simulink model "W01_Base_Map_cs"  (R2019a)
settings: Solver=FixedStepDiscrete  StartTime=0.0  StopTime=inf  FixedStep=1/20  RelTol=1e-3
PreLoadFcn:
  | mbxruntime.callbacks.PreLoadFcn(bdroot);
  | check_NUTS_defined
  | model_closed = 0;
  | assignin('base',['model_closed_' bdroot],false);
PostLoadFcn:
  | mbxruntime.callbacks.PostLoadFcn(bdroot);
InitFcn:
  | mbxruntime.callbacks.InitFcn(bdroot);
StartFcn:
  | mbxruntime.callbacks.StartFcn(bdroot);
StopFcn:
  | mbxruntime.callbacks.StopFcn(bdroot);;
  | 
model workspace: external: MAT-File .\W01_Base_Map_cs_hws.mat (data not in the file)
undefined symbols (not defined in the file or in its folder): DiscIntNeverNeededParam, Header, InitImageOutputDir, mbxruntime, Poses, Poses_SL_Info, tabledata, W01_Base_Map_cs_004987d4dd39f9b6, W01_Base_Map_cs_00cc66853e964a64, W01_Base_Map_cs_00f75b713170549a, W01_Base_Map_cs_01472650a6655f66, W01_Base_Map_cs_021eada97d6d5412, W01_Base_Map_cs_0288936122941f67, W01_Base_Map_cs_03728bc5c0f611d1, W01_Base_Map_cs_03729b7883682eca, W01_Base_Map_cs_03935175e827b825, W01_Base_Map_cs_03ecb5a7ceaf36f1, W01_Base_Map_cs_04544dd62153117c, W01_Base_Map_cs_04f0838a8dce3a91, W01_Base_Map_cs_05c6883b663017e6, W01_Base_Map_cs_074ff6b44c8e4b42, W01_Base_Map_cs_0850adb5f9b52847, W01_Base_Map_cs_09b4416d284a38c0, W01_Base_Map_cs_09f1a8cccf5dc476, W01_Base_Map_cs_0a863e6a78242047, W01_Base_Map_cs_0b51b2edfb6b21eb, W01_Base_Map_cs_0c25b2d8edd3fbea, W01_Base_Map_cs_0cec291d859792a3, W01_Base_Map_cs_0d48999ceb9def0a, W01_Base_Map_cs_1054e386bc2b89f8, W01_Base_Map_cs_129d7fd29679c9e4, W01_Base_Map_cs_1557dafebe6eb5e3, W01_Base_Map_cs_155bf6da17508b9f, W01_Base_Map_cs_1619aae3285d69a6, W01_Base_Map_cs_18faf784f59d6ded, W01_Base_Map_cs_190ae931cd3b3df1, W01_Base_Map_cs_1a47612a95ab18a1, W01_Base_Map_cs_1a96581334d27a16, W01_Base_Map_cs_1b9c28e1ad91b987, W01_Base_Map_cs_1bd80946b29cc249, W01_Base_Map_cs_1bf8c5472ecd97cc, W01_Base_Map_cs_1c047b8f6e9a46e9, W01_Base_Map_cs_1c4e91c4c8848966, W01_Base_Map_cs_1dfe629d3c3a34d6, W01_Base_Map_cs_1e00e80d4fa95f87, W01_Base_Map_cs_1e67a7d0e7e33a10, W01_Base_Map_cs_1e994bb86296e53e, W01_Base_Map_cs_1f3d28b65a209a81, W01_Base_Map_cs_1f4ddfcaed2bdfa2, W01_Base_Map_cs_20e6a062a8bf989a, W01_Base_Map_cs_210ba2feda70a68e, W01_Base_Map_cs_211f71a4af886b52, W01_Base_Map_cs_2177d1459a678375, W01_Base_Map_cs_21a90c8036f5a434, W01_Base_Map_cs_230365adf03440eb, W01_Base_Map_cs_2309b1b7588d9eb5, W01_Base_Map_cs_25766054964f8b23, W01_Base_Map_cs_25e42a2c513fe98c, W01_Base_Map_cs_25e53e1123ccd658, W01_Base_Map_cs_263f0dd851f19fdf ... (+283)
libraries: PreScanSimulinkLibrary x112, robotcorelib x55, adeye_lib x46, simulink x31, simulink_extras x24, robotlib x3, PreScanUsefulBlocks x1
(part 21 of 32)

== system W01_Base_Map_cs/Male_LargeShoulderSuitcase_1/SELF_Demux ==
  SELF : Inport  OutDataTypeStr=Bus: PRESCAN_SELFSENSORDATA
  Bus Selector : BusSelector  OutputSignals=PositionX,PositionY,PositionZ,OrientationRoll,OrientationPitch,OrientationYaw,Velocity,Yaw_rate,Lat,Long,Alt,TimeStamp
  Demux2 : Demux  Outputs=3
  Gain : Gain  Gain=180/pi
  Gain1 : Gain  Gain=180/pi
  Vector Concatenate1 : Concatenate  NumInputs=3
  compas converter : Subsystem
  x [m] : Outport
  y [m] : Outport  Port=2
  z [m] : Outport  Port=3
  rotx [deg] : Outport  Port=4
  roty [deg] : Outport  Port=5
  rotz [deg] : Outport  Port=6
  GPS lat [deg] : Outport  Port=7
  GPS long [deg] : Outport  Port=8
  GPS alt [m] : Outport  Port=9
  velocity [m/s] : Outport  Port=10
  heading [deg] : Outport  Port=11
  yaw rate [deg/s] : Outport  Port=12
  TimeStamp [s] : Outport  Port=13
  wires:
  Bus Selector/12 -> TimeStamp [s]/1  "<TimeStamp>"
  Bus Selector/11 -> GPS alt [m]/1  "<Alt>"
  Bus Selector/10 -> GPS long [deg]/1  "<Long>"
  Bus Selector/9 -> GPS lat [deg]/1  "<Lat>"
  Bus Selector/8 -> Gain1/1  "<Yaw_rate>"
  Bus Selector/7 -> velocity [m/s]/1  "<Velocity>"
  Bus Selector/6 -> compas converter/1(rotz [rad]), Vector Concatenate1/3  "<OrientationYaw>"
  Bus Selector/5 -> Vector Concatenate1/2  "<OrientationPitch>"
  Bus Selector/4 -> Vector Concatenate1/1  "<OrientationRoll>"
  Vector Concatenate1/1 -> Gain/1
  Bus Selector/3 -> z [m]/1  "<PositionZ>"
  Bus Selector/2 -> y [m]/1  "<PositionY>"
  Bus Selector/1 -> x [m]/1  "<PositionX>"
  SELF/1 -> Bus Selector/1
  Gain/1 -> Demux2/1
  Demux2/1 -> rotx [deg]/1
  Demux2/2 -> roty [deg]/1
  Demux2/3 -> rotz [deg]/1
  compas converter/1(heading [deg]) -> heading [deg]/1
  Gain1/1 -> yaw rate [deg/s]/1

== system W01_Base_Map_cs/Male_LargeShoulderSuitcase_1/VISUColorRegion_Bag_Mux ==
  RGB [-,-,-] : Inport
  Bus Creator : BusCreator  Inputs=4  OutDataTypeStr=Bus: PRESCAN_COLOR_DATA  NonVirtualBus=on
  Constant : Constant  Value=255  OutDataTypeStr=uint8
  Data Type Conversion : DataTypeConversion  OutDataTypeStr=uint8
  Data Type Conversion1 : DataTypeConversion  OutDataTypeStr=uint8
  Data Type Conversion2 : DataTypeConversion  OutDataTypeStr=uint8
  Demux : Demux  Outputs=3
  ColorRegion : Outport  OutDataTypeStr=Bus: PRESCAN_COLOR_DATA  PortDimensions=1
  wires:
  Constant/1 -> Bus Creator/4  "A"
  Data Type Conversion2/1 -> Bus Creator/3  "B"
  Data Type Conversion1/1 -> Bus Creator/2  "G"
  Data Type Conversion/1 -> Bus Creator/1  "R"
  Demux/3 -> Data Type Conversion2/1  "B"
  Demux/2 -> Data Type Conversion1/1  "G"
  Demux/1 -> Data Type Conversion/1  "R"
  RGB [-,-,-]/1 -> Demux/1
  Bus Creator/1 -> ColorRegion/1

== system W01_Base_Map_cs/Male_LargeShoulderSuitcase_1/VISUColorRegion_Lower_Body_Mux ==
  RGB [-,-,-] : Inport
  Bus Creator : BusCreator  Inputs=4  OutDataTypeStr=Bus: PRESCAN_COLOR_DATA  NonVirtualBus=on
  Constant : Constant  Value=255  OutDataTypeStr=uint8
  Data Type Conversion : DataTypeConversion  OutDataTypeStr=uint8
  Data Type Conversion1 : DataTypeConversion  OutDataTypeStr=uint8
  Data Type Conversion2 : DataTypeConversion  OutDataTypeStr=uint8
  Demux : Demux  Outputs=3
  ColorRegion : Outport  OutDataTypeStr=Bus: PRESCAN_COLOR_DATA  PortDimensions=1
  wires:
  Constant/1 -> Bus Creator/4  "A"
  Data Type Conversion2/1 -> Bus Creator/3  "B"
  Data Type Conversion1/1 -> Bus Creator/2  "G"
  Data Type Conversion/1 -> Bus Creator/1  "R"
  Demux/3 -> Data Type Conversion2/1  "B"
  Demux/2 -> Data Type Conversion1/1  "G"
  Demux/1 -> Data Type Conversion/1  "R"
  RGB [-,-,-]/1 -> Demux/1
  Bus Creator/1 -> ColorRegion/1

== system W01_Base_Map_cs/Male_LargeShoulderSuitcase_1/VISUColorRegion_Shoes_Mux ==
  RGB [-,-,-] : Inport
  Bus Creator : BusCreator  Inputs=4  OutDataTypeStr=Bus: PRESCAN_COLOR_DATA  NonVirtualBus=on
  Constant : Constant  Value=255  OutDataTypeStr=uint8
  Data Type Conversion : DataTypeConversion  OutDataTypeStr=uint8
  Data Type Conversion1 : DataTypeConversion  OutDataTypeStr=uint8
  Data Type Conversion2 : DataTypeConversion  OutDataTypeStr=uint8
  Demux : Demux  Outputs=3
  ColorRegion : Outport  OutDataTypeStr=Bus: PRESCAN_COLOR_DATA  PortDimensions=1
  wires:
  Constant/1 -> Bus Creator/4  "A"
  Data Type Conversion2/1 -> Bus Creator/3  "B"
  Data Type Conversion1/1 -> Bus Creator/2  "G"
  Data Type Conversion/1 -> Bus Creator/1  "R"
  Demux/3 -> Data Type Conversion2/1  "B"
  Demux/2 -> Data Type Conversion1/1  "G"
  Demux/1 -> Data Type Conversion/1  "R"
  RGB [-,-,-]/1 -> Demux/1
  Bus Creator/1 -> ColorRegion/1

== system W01_Base_Map_cs/Male_LargeShoulderSuitcase_1/VISUColorRegion_Upper_body_Mux ==
  RGB [-,-,-] : Inport
  Bus Creator : BusCreator  Inputs=4  OutDataTypeStr=Bus: PRESCAN_COLOR_DATA  NonVirtualBus=on
  Constant : Constant  Value=255  OutDataTypeStr=uint8
  Data Type Conversion : DataTypeConversion  OutDataTypeStr=uint8
  Data Type Conversion1 : DataTypeConversion  OutDataTypeStr=uint8
  Data Type Conversion2 : DataTypeConversion  OutDataTypeStr=uint8
  Demux : Demux  Outputs=3
  ColorRegion : Outport  OutDataTypeStr=Bus: PRESCAN_COLOR_DATA  PortDimensions=1
  wires:
  Constant/1 -> Bus Creator/4  "A"
  Data Type Conversion2/1 -> Bus Creator/3  "B"
  Data Type Conversion1/1 -> Bus Creator/2  "G"
  Data Type Conversion/1 -> Bus Creator/1  "R"
  Demux/3 -> Data Type Conversion2/1  "B"
  Demux/2 -> Data Type Conversion1/1  "G"
  Demux/1 -> Data Type Conversion/1  "R"
  RGB [-,-,-]/1 -> Demux/1
  Bus Creator/1 -> ColorRegion/1

== system W01_Base_Map_cs/Male_Old_White_WithStick_1/Dynamics_Empty ==
  note: For state mode 'Dynamic' positions
      | are not taken into account, as they
      | are computed by integrating velocity.
      | Click annotation for Help.
  In1 : Inport
  Bus Creator : BusCreator  Inputs=3
  Bus Creator1 : BusCreator  Inputs=4
  Bus Selector : BusSelector  OutputSignals=signal1,signal2,signal3
  Bus Selector1 : BusSelector  OutputSignals=Pose.Position.X,Pose.Position.Y,Pose.Position.Z,Pose.Orientation.W,Pose.Orientation.X,Pose.Orientation.Y,Pose.Orientation.Z
  Bus to Vector : BusToVector
  Coordinate Transformation Conversion : robotcorelib/Coordinate Transformation Conversion  InputRepresentation=Quaternion  InputEulerSequence=ZYX  ShowTrVecInputPort=on  OutputRepresentation=Euler Angles  OutputEulerSequence=ZYX  ShowTrVecOutputPort=on  SimulateUsing=Interpreted execution
      settings: SourceProductBaseCode=RO
  Demux : Demux  Outputs=3
  Display{,1..3} (4 alike) : Display
  Ground_2 : Ground
  Ground_3 : Ground
  Ground_4 : Ground
  MuxState : Subsystem  Tag=mux/State  mask(Empty Dynamics State Block){positioningmode=on, TimeStep=1/20}
      mask prompts: positioningmode "Positioning Mode"; TimeStep "Auto Assigned: Time Step [s]"
      mask help:
      | Build the state of an actor based on user input.
      | The user can either use positioning mode or dynamics mode.
      | - When using positioning mode the position and orientation of the actor are set directly based on the input. Expected input is relative to the initial position and orientation of the actor. It's also possible to specify the velocity of the actor, though this input isn't used, only passed on.
      | - When using dynamics mode the position input is ignored. Expected input is velocity and orientation. The velocity is relative the current orientation of the actor, while orientation is relative to its initial orientation. The position of the actor is calculated based on the velocity and orientation given.
      settings: DeleteFcn=PreScanBlockDeleteFcn;
  STATE_Male_Old_White_WithStick_1 : Subsystem  Tag=mux/StatePort  Priority=0  LoadFcn=load PrescanStateActuatorData  mask(PreScan Sink Block: State){x0=W01_Base_Map_cs_cc1dceb6bcb11776, y0=W01_Base_Map_cs_dd1c45dbea022fa7, z0=W01_Base_Map_cs_395a0412cd743ae4, Roll0=W01_Base_Map_cs_f8d27bdcf4af038a, Pitch0=W01_Base_Map_cs_2bee40668d322807, Yaw0=W01_Base_Map_cs_3225b4cbe8940148, TimeStep=1/20}
      mask prompts: x0 "Ini x-position VEHICLE wrt GLOBAL axis system [m]"; y0 "Ini y-position VEHICLE wrt GLOBAL axis system [m]"; z0 "Ini z-position VEHICLE wrt GLOBAL axis system [m]"; Roll0 "Ini roll-angle BODY wrt VEHICLE axis system [deg]"; Pitch0 "Ini pitch-angle BODY wrt VEHICLE axis system [deg]"; Yaw0 "Ini yaw-angle VEHICLE wrt GLOBAL axis system [deg]"; TimeStep "Auto-Assigned: Upload Period [s]"
      mask help:
      | The Actor State contains a vector signal of size (9x1), containing the following signals:
      |
      | -  Position                  (x,y,z)                                     [m]
      | -  Velocity                  (vx,vy,vz)                               [m/s]
      | -  Angles                    (Roll, Pitch, Yaw)                   [rad]
      |
      | The Actor state is defined in the global axis system.
      | The state is superponed on the Initial position defined in the GUI.
      |
      | For more information, please click Help.
      settings: DeleteFcn=PreScanBlockDeleteFcn;
      mask Help: eval('openHelp(222)')
      mask Display: image(imread('State.png'))
  To Virtual Bus : SignalConversion  ConversionOutput=Virtual bus  OverrideOpt=off
  State : Outport  Tag=outport/StateOutport  SampleTime=1/20
  wires:
  MuxState/1(state) -> STATE_Male_Old_White_WithStick_1/1(State)
  STATE_Male_Old_White_WithStick_1/1(StateBus) -> State/1
  Ground_2/1 -> MuxState/4(dx [m/s])
  Ground_3/1 -> MuxState/5(dy [m/s])
  Ground_4/1 -> MuxState/6(dz [m/s])
  Bus Selector/2 -> MuxState/8(P [rad]), Display/1  "<signal2>"
  Bus Selector/1 -> MuxState/7(R [rad]), Display2/1  "<signal1>"
  Bus Selector1/2 -> MuxState/2(y [m])  "<Y>"
  Bus Selector1/1 -> MuxState/1(x [m])  "<X>"
  Coordinate Transformation Conversion/1 -> Demux/1
  Demux/1 -> Bus Creator/1
  To Virtual Bus/1 -> Bus to Vector/1
  In1/1 -> Bus Selector1/1
  Bus to Vector/1 -> Display3/1, Coordinate Transformation Conversion/1
  Bus Creator1/1 -> To Virtual Bus/1
  Demux/2 -> Bus Creator/2
  Demux/3 -> Bus Creator/3
  Bus Creator/1 -> Bus Selector/1
  Bus Selector1/7 -> Bus Creator1/4  "<Z>"
  Bus Selector1/4 -> Bus Creator1/1  "<W>"
  Bus Selector/3 -> MuxState/9(Y [rad]), Display1/1  "<signal3>"
  Bus Selector1/5 -> Bus Creator1/2  "<X>"
  Bus Selector1/3 -> MuxState/3(z [m])  "<Z>"
  Bus Selector1/6 -> Bus Creator1/3  "<Y>"

== system W01_Base_Map_cs/Male_Old_White_WithStick_1/SELF_Demux ==
  SELF : Inport  OutDataTypeStr=Bus: PRESCAN_SELFSENSORDATA
  Bus Selector : BusSelector  OutputSignals=PositionX,PositionY,PositionZ,OrientationRoll,OrientationPitch,OrientationYaw,Velocity,Yaw_rate,Lat,Long,Alt,TimeStamp
  Demux2 : Demux  Outputs=3
  Gain : Gain  Gain=180/pi
  Gain1 : Gain  Gain=180/pi
  Vector Concatenate1 : Concatenate  NumInputs=3
  compas converter : Subsystem
  x [m] : Outport
  y [m] : Outport  Port=2
  z [m] : Outport  Port=3
  rotx [deg] : Outport  Port=4
  roty [deg] : Outport  Port=5
  rotz [deg] : Outport  Port=6
  GPS lat [deg] : Outport  Port=7
  GPS long [deg] : Outport  Port=8
  GPS alt [m] : Outport  Port=9
  velocity [m/s] : Outport  Port=10
  heading [deg] : Outport  Port=11
  yaw rate [deg/s] : Outport  Port=12
  TimeStamp [s] : Outport  Port=13
  wires:
  Bus Selector/12 -> TimeStamp [s]/1  "<TimeStamp>"
  Bus Selector/11 -> GPS alt [m]/1  "<Alt>"
  Bus Selector/10 -> GPS long [deg]/1  "<Long>"
  Bus Selector/9 -> GPS lat [deg]/1  "<Lat>"
  Bus Selector/8 -> Gain1/1  "<Yaw_rate>"
  Bus Selector/7 -> velocity [m/s]/1  "<Velocity>"
  Bus Selector/6 -> compas converter/1(rotz [rad]), Vector Concatenate1/3  "<OrientationYaw>"
  Bus Selector/5 -> Vector Concatenate1/2  "<OrientationPitch>"
  Bus Selector/4 -> Vector Concatenate1/1  "<OrientationRoll>"
  Vector Concatenate1/1 -> Gain/1
  Bus Selector/3 -> z [m]/1  "<PositionZ>"
  Bus Selector/2 -> y [m]/1  "<PositionY>"
  Bus Selector/1 -> x [m]/1  "<PositionX>"
  SELF/1 -> Bus Selector/1
  Gain/1 -> Demux2/1
  Demux2/1 -> rotx [deg]/1
  Demux2/2 -> roty [deg]/1
  Demux2/3 -> rotz [deg]/1
  compas converter/1(heading [deg]) -> heading [deg]/1
  Gain1/1 -> yaw rate [deg/s]/1

== system W01_Base_Map_cs/Male_Old_White_WithStick_1/VISUColorRegion_Lower_Body_Mux ==
  RGB [-,-,-] : Inport
  Bus Creator : BusCreator  Inputs=4  OutDataTypeStr=Bus: PRESCAN_COLOR_DATA  NonVirtualBus=on
  Constant : Constant  Value=255  OutDataTypeStr=uint8
  Data Type Conversion : DataTypeConversion  OutDataTypeStr=uint8
  Data Type Conversion1 : DataTypeConversion  OutDataTypeStr=uint8
  Data Type Conversion2 : DataTypeConversion  OutDataTypeStr=uint8
  Demux : Demux  Outputs=3
  ColorRegion : Outport  OutDataTypeStr=Bus: PRESCAN_COLOR_DATA  PortDimensions=1
  wires:
  Constant/1 -> Bus Creator/4  "A"
  Data Type Conversion2/1 -> Bus Creator/3  "B"
  Data Type Conversion1/1 -> Bus Creator/2  "G"
  Data Type Conversion/1 -> Bus Creator/1  "R"
  Demux/3 -> Data Type Conversion2/1  "B"
  Demux/2 -> Data Type Conversion1/1  "G"
  Demux/1 -> Data Type Conversion/1  "R"
  RGB [-,-,-]/1 -> Demux/1
  Bus Creator/1 -> ColorRegion/1

== system W01_Base_Map_cs/Male_Old_White_WithStick_1/VISUColorRegion_Shoes_Mux ==
  RGB [-,-,-] : Inport
  Bus Creator : BusCreator  Inputs=4  OutDataTypeStr=Bus: PRESCAN_COLOR_DATA  NonVirtualBus=on
  Constant : Constant  Value=255  OutDataTypeStr=uint8
  Data Type Conversion : DataTypeConversion  OutDataTypeStr=uint8
  Data Type Conversion1 : DataTypeConversion  OutDataTypeStr=uint8
  Data Type Conversion2 : DataTypeConversion  OutDataTypeStr=uint8
  Demux : Demux  Outputs=3
  ColorRegion : Outport  OutDataTypeStr=Bus: PRESCAN_COLOR_DATA  PortDimensions=1
  wires:
  Constant/1 -> Bus Creator/4  "A"
  Data Type Conversion2/1 -> Bus Creator/3  "B"
  Data Type Conversion1/1 -> Bus Creator/2  "G"
  Data Type Conversion/1 -> Bus Creator/1  "R"
  Demux/3 -> Data Type Conversion2/1  "B"
  Demux/2 -> Data Type Conversion1/1  "G"
  Demux/1 -> Data Type Conversion/1  "R"
  RGB [-,-,-]/1 -> Demux/1
  Bus Creator/1 -> ColorRegion/1

== system W01_Base_Map_cs/Male_Old_White_WithStick_1/VISUColorRegion_Upper_Body_Mux ==
  RGB [-,-,-] : Inport
  Bus Creator : BusCreator  Inputs=4  OutDataTypeStr=Bus: PRESCAN_COLOR_DATA  NonVirtualBus=on
  Constant : Constant  Value=255  OutDataTypeStr=uint8
  Data Type Conversion : DataTypeConversion  OutDataTypeStr=uint8
  Data Type Conversion1 : DataTypeConversion  OutDataTypeStr=uint8
  Data Type Conversion2 : DataTypeConversion  OutDataTypeStr=uint8
  Demux : Demux  Outputs=3
  ColorRegion : Outport  OutDataTypeStr=Bus: PRESCAN_COLOR_DATA  PortDimensions=1
  wires:
  Constant/1 -> Bus Creator/4  "A"
  Data Type Conversion2/1 -> Bus Creator/3  "B"
  Data Type Conversion1/1 -> Bus Creator/2  "G"
  Data Type Conversion/1 -> Bus Creator/1  "R"
  Demux/3 -> Data Type Conversion2/1  "B"
  Demux/2 -> Data Type Conversion1/1  "G"
  Demux/1 -> Data Type Conversion/1  "R"
  RGB [-,-,-]/1 -> Demux/1
  Bus Creator/1 -> ColorRegion/1

== system W01_Base_Map_cs/Male_Old_White_WithWalkerWithWheels_1/Dynamics_Empty ==
  note: For state mode 'Dynamic' positions
      | are not taken into account, as they
      | are computed by integrating velocity.
      | Click annotation for Help.
  In1 : Inport
  Bus Creator : BusCreator  Inputs=3
  Bus Creator1 : BusCreator  Inputs=4
  Bus Selector : BusSelector  OutputSignals=signal1,signal2,signal3
  Bus Selector1 : BusSelector  OutputSignals=Pose.Position.X,Pose.Position.Y,Pose.Position.Z,Pose.Orientation.W,Pose.Orientation.X,Pose.Orientation.Y,Pose.Orientation.Z
  Bus to Vector : BusToVector
  Coordinate Transformation Conversion : robotcorelib/Coordinate Transformation Conversion  InputRepresentation=Quaternion  InputEulerSequence=ZYX  ShowTrVecInputPort=on  OutputRepresentation=Euler Angles  OutputEulerSequence=ZYX  ShowTrVecOutputPort=on  SimulateUsing=Interpreted execution
      settings: SourceProductBaseCode=RO
  Demux : Demux  Outputs=3
  Display{,1..3} (4 alike) : Display
  Ground_2 : Ground
  Ground_3 : Ground
  Ground_4 : Ground
  MuxState : Subsystem  Tag=mux/State  mask(Empty Dynamics State Block){positioningmode=on, TimeStep=1/20}
      mask prompts: positioningmode "Positioning Mode"; TimeStep "Auto Assigned: Time Step [s]"
      mask help:
      | Build the state of an actor based on user input.
      | The user can either use positioning mode or dynamics mode.
      | - When using positioning mode the position and orientation of the actor are set directly based on the input. Expected input is relative to the initial position and orientation of the actor. It's also possible to specify the velocity of the actor, though this input isn't used, only passed on.
      | - When using dynamics mode the position input is ignored. Expected input is velocity and orientation. The velocity is relative the current orientation of the actor, while orientation is relative to its initial orientation. The position of the actor is calculated based on the velocity and orientation given.
      settings: DeleteFcn=PreScanBlockDeleteFcn;
  STATE_Male_Old_White_WithWalkerWithWheels_1 : Subsystem  Tag=mux/StatePort  Priority=0  LoadFcn=load PrescanStateActuatorData  mask(PreScan Sink Block: State){x0=W01_Base_Map_cs_55eb73129df87210, y0=W01_Base_Map_cs_bf64c7ba95b0aa28, z0=W01_Base_Map_cs_34d2d6374cf9c3dd, Roll0=W01_Base_Map_cs_01472650a6655f66, Pitch0=W01_Base_Map_cs_7cad10af2de5dd89, Yaw0=W01_Base_Map_cs_fd671e9618ff8c80, TimeStep=1/20}
      mask prompts: x0 "Ini x-position VEHICLE wrt GLOBAL axis system [m]"; y0 "Ini y-position VEHICLE wrt GLOBAL axis system [m]"; z0 "Ini z-position VEHICLE wrt GLOBAL axis system [m]"; Roll0 "Ini roll-angle BODY wrt VEHICLE axis system [deg]"; Pitch0 "Ini pitch-angle BODY wrt VEHICLE axis system [deg]"; Yaw0 "Ini yaw-angle VEHICLE wrt GLOBAL axis system [deg]"; TimeStep "Auto-Assigned: Upload Period [s]"
      mask help:
      | The Actor State contains a vector signal of size (9x1), containing the following signals:
      |
      | -  Position                  (x,y,z)                                     [m]
      | -  Velocity                  (vx,vy,vz)                               [m/s]
      | -  Angles                    (Roll, Pitch, Yaw)                   [rad]
      |
      | The Actor state is defined in the global axis system.
      | The state is superponed on the Initial position defined in the GUI.
      |
      | For more information, please click Help.
      settings: DeleteFcn=PreScanBlockDeleteFcn;
      mask Help: eval('openHelp(222)')
      mask Display: image(imread('State.png'))
  To Virtual Bus : SignalConversion  ConversionOutput=Virtual bus  OverrideOpt=off
  State : Outport  Tag=outport/StateOutport  SampleTime=1/20
  wires:
  MuxState/1(state) -> STATE_Male_Old_White_WithWalkerWithWheels_1/1(State)
  STATE_Male_Old_White_WithWalkerWithWheels_1/1(StateBus) -> State/1
  Ground_2/1 -> MuxState/4(dx [m/s])
  Ground_3/1 -> MuxState/5(dy [m/s])
  Ground_4/1 -> MuxState/6(dz [m/s])
  Bus Selector/2 -> MuxState/8(P [rad]), Display/1  "<signal2>"
  Bus Selector/1 -> MuxState/7(R [rad]), Display2/1  "<signal1>"
  Bus Selector1/2 -> MuxState/2(y [m])  "<Y>"
  Bus Selector1/1 -> MuxState/1(x [m])  "<X>"
  Coordinate Transformation Conversion/1 -> Demux/1
  Demux/1 -> Bus Creator/1
  To Virtual Bus/1 -> Bus to Vector/1
  In1/1 -> Bus Selector1/1
  Bus to Vector/1 -> Display3/1, Coordinate Transformation Conversion/1
  Bus Creator1/1 -> To Virtual Bus/1
  Demux/2 -> Bus Creator/2
  Demux/3 -> Bus Creator/3
  Bus Creator/1 -> Bus Selector/1
  Bus Selector1/7 -> Bus Creator1/4  "<Z>"
  Bus Selector1/4 -> Bus Creator1/1  "<W>"
  Bus Selector/3 -> MuxState/9(Y [rad]), Display1/1  "<signal3>"
  Bus Selector1/5 -> Bus Creator1/2  "<X>"
  Bus Selector1/3 -> MuxState/3(z [m])  "<Z>"
  Bus Selector1/6 -> Bus Creator1/3  "<Y>"

== system W01_Base_Map_cs/Male_Old_White_WithWalkerWithWheels_1/SELF_Demux ==
  SELF : Inport  OutDataTypeStr=Bus: PRESCAN_SELFSENSORDATA
  Bus Selector : BusSelector  OutputSignals=PositionX,PositionY,PositionZ,OrientationRoll,OrientationPitch,OrientationYaw,Velocity,Yaw_rate,Lat,Long,Alt,TimeStamp
  Demux2 : Demux  Outputs=3
  Gain : Gain  Gain=180/pi
  Gain1 : Gain  Gain=180/pi
  Vector Concatenate1 : Concatenate  NumInputs=3
  compas converter : Subsystem
  x [m] : Outport
  y [m] : Outport  Port=2
  z [m] : Outport  Port=3
  rotx [deg] : Outport  Port=4
  roty [deg] : Outport  Port=5
  rotz [deg] : Outport  Port=6
  GPS lat [deg] : Outport  Port=7
  GPS long [deg] : Outport  Port=8
  GPS alt [m] : Outport  Port=9
  velocity [m/s] : Outport  Port=10
  heading [deg] : Outport  Port=11
  yaw rate [deg/s] : Outport  Port=12
  TimeStamp [s] : Outport  Port=13
  wires:
  Bus Selector/12 -> TimeStamp [s]/1  "<TimeStamp>"
  Bus Selector/11 -> GPS alt [m]/1  "<Alt>"
  Bus Selector/10 -> GPS long [deg]/1  "<Long>"
  Bus Selector/9 -> GPS lat [deg]/1  "<Lat>"
  Bus Selector/8 -> Gain1/1  "<Yaw_rate>"
  Bus Selector/7 -> velocity [m/s]/1  "<Velocity>"
  Bus Selector/6 -> compas converter/1(rotz [rad]), Vector Concatenate1/3  "<OrientationYaw>"
  Bus Selector/5 -> Vector Concatenate1/2  "<OrientationPitch>"
  Bus Selector/4 -> Vector Concatenate1/1  "<OrientationRoll>"
  Vector Concatenate1/1 -> Gain/1
  Bus Selector/3 -> z [m]/1  "<PositionZ>"
  Bus Selector/2 -> y [m]/1  "<PositionY>"
  Bus Selector/1 -> x [m]/1  "<PositionX>"
  SELF/1 -> Bus Selector/1
  Gain/1 -> Demux2/1
  Demux2/1 -> rotx [deg]/1
  Demux2/2 -> roty [deg]/1
  Demux2/3 -> rotz [deg]/1
  compas converter/1(heading [deg]) -> heading [deg]/1
  Gain1/1 -> yaw rate [deg/s]/1

== system W01_Base_Map_cs/Male_Old_White_WithWalkerWithWheels_1/VISUColorRegion_Lower_Body_Mux ==
  RGB [-,-,-] : Inport
  Bus Creator : BusCreator  Inputs=4  OutDataTypeStr=Bus: PRESCAN_COLOR_DATA  NonVirtualBus=on
  Constant : Constant  Value=255  OutDataTypeStr=uint8
  Data Type Conversion : DataTypeConversion  OutDataTypeStr=uint8
  Data Type Conversion1 : DataTypeConversion  OutDataTypeStr=uint8
  Data Type Conversion2 : DataTypeConversion  OutDataTypeStr=uint8
  Demux : Demux  Outputs=3
  ColorRegion : Outport  OutDataTypeStr=Bus: PRESCAN_COLOR_DATA  PortDimensions=1
  wires:
  Constant/1 -> Bus Creator/4  "A"
  Data Type Conversion2/1 -> Bus Creator/3  "B"
  Data Type Conversion1/1 -> Bus Creator/2  "G"
  Data Type Conversion/1 -> Bus Creator/1  "R"
  Demux/3 -> Data Type Conversion2/1  "B"
  Demux/2 -> Data Type Conversion1/1  "G"
  Demux/1 -> Data Type Conversion/1  "R"
  RGB [-,-,-]/1 -> Demux/1
  Bus Creator/1 -> ColorRegion/1

== system W01_Base_Map_cs/Male_Old_White_WithWalkerWithWheels_1/VISUColorRegion_Shoes_Mux ==
  RGB [-,-,-] : Inport
  Bus Creator : BusCreator  Inputs=4  OutDataTypeStr=Bus: PRESCAN_COLOR_DATA  NonVirtualBus=on
  Constant : Constant  Value=255  OutDataTypeStr=uint8
  Data Type Conversion : DataTypeConversion  OutDataTypeStr=uint8
  Data Type Conversion1 : DataTypeConversion  OutDataTypeStr=uint8
  Data Type Conversion2 : DataTypeConversion  OutDataTypeStr=uint8
  Demux : Demux  Outputs=3
  ColorRegion : Outport  OutDataTypeStr=Bus: PRESCAN_COLOR_DATA  PortDimensions=1
  wires:
  Constant/1 -> Bus Creator/4  "A"
  Data Type Conversion2/1 -> Bus Creator/3  "B"
  Data Type Conversion1/1 -> Bus Creator/2  "G"
  Data Type Conversion/1 -> Bus Creator/1  "R"
  Demux/3 -> Data Type Conversion2/1  "B"
  Demux/2 -> Data Type Conversion1/1  "G"
  Demux/1 -> Data Type Conversion/1  "R"
  RGB [-,-,-]/1 -> Demux/1
  Bus Creator/1 -> ColorRegion/1

== system W01_Base_Map_cs/Male_Old_White_WithWalkerWithWheels_1/VISUColorRegion_Upper_Body_Mux ==
  RGB [-,-,-] : Inport
  Bus Creator : BusCreator  Inputs=4  OutDataTypeStr=Bus: PRESCAN_COLOR_DATA  NonVirtualBus=on
  Constant : Constant  Value=255  OutDataTypeStr=uint8
  Data Type Conversion : DataTypeConversion  OutDataTypeStr=uint8
  Data Type Conversion1 : DataTypeConversion  OutDataTypeStr=uint8
  Data Type Conversion2 : DataTypeConversion  OutDataTypeStr=uint8
  Demux : Demux  Outputs=3
  ColorRegion : Outport  OutDataTypeStr=Bus: PRESCAN_COLOR_DATA  PortDimensions=1
  wires:
  Constant/1 -> Bus Creator/4  "A"
  Data Type Conversion2/1 -> Bus Creator/3  "B"
  Data Type Conversion1/1 -> Bus Creator/2  "G"
  Data Type Conversion/1 -> Bus Creator/1  "R"
  Demux/3 -> Data Type Conversion2/1  "B"
  Demux/2 -> Data Type Conversion1/1  "G"
  Demux/1 -> Data Type Conversion/1  "R"
  RGB [-,-,-]/1 -> Demux/1
  Bus Creator/1 -> ColorRegion/1

== system W01_Base_Map_cs/Male_Old_White_WithWalker_1/Dynamics_Empty ==
  note: For state mode 'Dynamic' positions
      | are not taken into account, as they
      | are computed by integrating velocity.
      | Click annotation for Help.
  In1 : Inport
  Bus Creator : BusCreator  Inputs=3
  Bus Creator1 : BusCreator  Inputs=4
  Bus Selector : BusSelector  OutputSignals=signal1,signal2,signal3
  Bus Selector1 : BusSelector  OutputSignals=Pose.Position.X,Pose.Position.Y,Pose.Position.Z,Pose.Orientation.W,Pose.Orientation.X,Pose.Orientation.Y,Pose.Orientation.Z
  Bus to Vector : BusToVector
  Coordinate Transformation Conversion : robotcorelib/Coordinate Transformation Conversion  InputRepresentation=Quaternion  InputEulerSequence=ZYX  ShowTrVecInputPort=on  OutputRepresentation=Euler Angles  OutputEulerSequence=ZYX  ShowTrVecOutputPort=on  SimulateUsing=Interpreted execution
      settings: SourceProductBaseCode=RO
  Demux : Demux  Outputs=3
  Display{,1..3} (4 alike) : Display
  Ground_2 : Ground
  Ground_3 : Ground
  Ground_4 : Ground
  MuxState : Subsystem  Tag=mux/State  mask(Empty Dynamics State Block){positioningmode=on, TimeStep=1/20}
      mask prompts: positioningmode "Positioning Mode"; TimeStep "Auto Assigned: Time Step [s]"
      mask help:
      | Build the state of an actor based on user input.
      | The user can either use positioning mode or dynamics mode.
      | - When using positioning mode the position and orientation of the actor are set directly based on the input. Expected input is relative to the initial position and orientation of the actor. It's also possible to specify the velocity of the actor, though this input isn't used, only passed on.
      | - When using dynamics mode the position input is ignored. Expected input is velocity and orientation. The velocity is relative the current orientation of the actor, while orientation is relative to its initial orientation. The position of the actor is calculated based on the velocity and orientation given.
      settings: DeleteFcn=PreScanBlockDeleteFcn;
  STATE_Male_Old_White_WithWalker_1 : Subsystem  Tag=mux/StatePort  Priority=0  LoadFcn=load PrescanStateActuatorData  mask(PreScan Sink Block: State){x0=W01_Base_Map_cs_263f0dd851f19fdf, y0=W01_Base_Map_cs_ca449718feba9361, z0=W01_Base_Map_cs_f3562cd5b7ad7352, Roll0=W01_Base_Map_cs_f448d0261a15344f, Pitch0=W01_Base_Map_cs_dacfbbbb8bc566f6, Yaw0=W01_Base_Map_cs_e5793aff7e695769, TimeStep=1/20}
      mask prompts: x0 "Ini x-position VEHICLE wrt GLOBAL axis system [m]"; y0 "Ini y-position VEHICLE wrt GLOBAL axis system [m]"; z0 "Ini z-position VEHICLE wrt GLOBAL axis system [m]"; Roll0 "Ini roll-angle BODY wrt VEHICLE axis system [deg]"; Pitch0 "Ini pitch-angle BODY wrt VEHICLE axis system [deg]"; Yaw0 "Ini yaw-angle VEHICLE wrt GLOBAL axis system [deg]"; TimeStep "Auto-Assigned: Upload Period [s]"
      mask help:
      | The Actor State contains a vector signal of size (9x1), containing the following signals:
      |
      | -  Position                  (x,y,z)                                     [m]
      | -  Velocity                  (vx,vy,vz)                               [m/s]
      | -  Angles                    (Roll, Pitch, Yaw)                   [rad]
      |
      | The Actor state is defined in the global axis system.
      | The state is superponed on the Initial position defined in the GUI.
      |
      | For more information, please click Help.
      settings: DeleteFcn=PreScanBlockDeleteFcn;
      mask Help: eval('openHelp(222)')
      mask Display: image(imread('State.png'))
  To Virtual Bus : SignalConversion  ConversionOutput=Virtual bus  OverrideOpt=off
  State : Outport  Tag=outport/StateOutport  SampleTime=1/20
  wires:
  MuxState/1(state) -> STATE_Male_Old_White_WithWalker_1/1(State)
  STATE_Male_Old_White_WithWalker_1/1(StateBus) -> State/1
  Ground_2/1 -> MuxState/4(dx [m/s])
  Ground_3/1 -> MuxState/5(dy [m/s])
  Ground_4/1 -> MuxState/6(dz [m/s])
  Bus Selector/2 -> MuxState/8(P [rad]), Display/1  "<signal2>"
  Bus Selector/1 -> MuxState/7(R [rad]), Display2/1  "<signal1>"
  Bus Selector1/2 -> MuxState/2(y [m])  "<Y>"
  Bus Selector1/1 -> MuxState/1(x [m])  "<X>"
  Coordinate Transformation Conversion/1 -> Demux/1
  Demux/1 -> Bus Creator/1
  To Virtual Bus/1 -> Bus to Vector/1
  Bus to Vector/1 -> Display3/1, Coordinate Transformation Conversion/1
  Bus Creator1/1 -> To Virtual Bus/1
  Demux/2 -> Bus Creator/2
  Demux/3 -> Bus Creator/3
  Bus Creator/1 -> Bus Selector/1
  Bus Selector1/7 -> Bus Creator1/4  "<Z>"
  Bus Selector1/4 -> Bus Creator1/1  "<W>"
  Bus Selector/3 -> MuxState/9(Y [rad]), Display1/1  "<signal3>"
  Bus Selector1/5 -> Bus Creator1/2  "<X>"
  Bus Selector1/3 -> MuxState/3(z [m])  "<Z>"
  Bus Selector1/6 -> Bus Creator1/3  "<Y>"
  In1/1 -> Bus Selector1/1

== system W01_Base_Map_cs/Male_Old_White_WithWalker_1/SELF_Demux ==
  SELF : Inport  OutDataTypeStr=Bus: PRESCAN_SELFSENSORDATA
  Bus Selector : BusSelector  OutputSignals=PositionX,PositionY,PositionZ,OrientationRoll,OrientationPitch,OrientationYaw,Velocity,Yaw_rate,Lat,Long,Alt,TimeStamp
  Demux2 : Demux  Outputs=3
  Gain : Gain  Gain=180/pi
  Gain1 : Gain  Gain=180/pi
  Vector Concatenate1 : Concatenate  NumInputs=3
  compas converter : Subsystem
  x [m] : Outport
  y [m] : Outport  Port=2
  z [m] : Outport  Port=3
  rotx [deg] : Outport  Port=4
  roty [deg] : Outport  Port=5
  rotz [deg] : Outport  Port=6
  GPS lat [deg] : Outport  Port=7
  GPS long [deg] : Outport  Port=8
  GPS alt [m] : Outport  Port=9
  velocity [m/s] : Outport  Port=10
  heading [deg] : Outport  Port=11
  yaw rate [deg/s] : Outport  Port=12
  TimeStamp [s] : Outport  Port=13
  wires:
  Bus Selector/12 -> TimeStamp [s]/1  "<TimeStamp>"
  Bus Selector/11 -> GPS alt [m]/1  "<Alt>"
  Bus Selector/10 -> GPS long [deg]/1  "<Long>"
  Bus Selector/9 -> GPS lat [deg]/1  "<Lat>"
  Bus Selector/8 -> Gain1/1  "<Yaw_rate>"
  Bus Selector/7 -> velocity [m/s]/1  "<Velocity>"
  Bus Selector/6 -> compas converter/1(rotz [rad]), Vector Concatenate1/3  "<OrientationYaw>"
  Bus Selector/5 -> Vector Concatenate1/2  "<OrientationPitch>"
  Bus Selector/4 -> Vector Concatenate1/1  "<OrientationRoll>"
  Vector Concatenate1/1 -> Gain/1
  Bus Selector/3 -> z [m]/1  "<PositionZ>"
  Bus Selector/2 -> y [m]/1  "<PositionY>"
  Bus Selector/1 -> x [m]/1  "<PositionX>"
  SELF/1 -> Bus Selector/1
  Gain/1 -> Demux2/1
  Demux2/1 -> rotx [deg]/1
  Demux2/2 -> roty [deg]/1
  Demux2/3 -> rotz [deg]/1
  compas converter/1(heading [deg]) -> heading [deg]/1
  Gain1/1 -> yaw rate [deg/s]/1

== system W01_Base_Map_cs/Male_Overweight_1/Animation ==
  In1 : Inport
  Bus Creator : BusCreator  Inputs=2  OutDataTypeStr=Bus: PRESCAN_ANIMACTUATORDATA  NonVirtualBus=on
  Bus Selector : BusSelector  OutputSignals=VelocityX,VelocityY,VelocityZ
  Mux : Mux  Inputs=3
  animation mode : Subsystem
  elapsed track : Subsystem
  Out1 : Outport
  wires:
  animation mode/1(mode) -> Bus Creator/1  "Index"
  Bus Creator/1 -> Out1/1
  In1/1 -> Bus Selector/1
  elapsed track/1(s) -> Bus Creator/2  "Time"
  Bus Selector/3 -> Mux/3  "<VelocityZ>"
  Bus Selector/2 -> Mux/2  "<VelocityY>"
  Bus Selector/1 -> Mux/1  "<VelocityX>"
  Mux/1 -> animation mode/1(vel), elapsed track/1(vel)

== system W01_Base_Map_cs/Male_Overweight_1/Dynamics_Empty ==
  note: For state mode 'Dynamic' positions
      | are not taken into account, as they
      | are computed by integrating velocity.
      | Click annotation for Help.
  In1 : Inport
  Bus Creator : BusCreator  Inputs=3
  Bus Creator1 : BusCreator  Inputs=4
  Bus Selector : BusSelector  OutputSignals=signal1,signal2,signal3
  Bus Selector1 : BusSelector  OutputSignals=Pose.Position.X,Pose.Position.Y,Pose.Position.Z,Pose.Orientation.W,Pose.Orientation.X,Pose.Orientation.Y,Pose.Orientation.Z
  Bus to Vector : BusToVector
  Coordinate Transformation Conversion : robotcorelib/Coordinate Transformation Conversion  InputRepresentation=Quaternion  InputEulerSequence=ZYX  ShowTrVecInputPort=on  OutputRepresentation=Euler Angles  OutputEulerSequence=ZYX  ShowTrVecOutputPort=on  SimulateUsing=Interpreted execution
      settings: SourceProductBaseCode=RO
  Demux : Demux  Outputs=3
  Display{,1..3} (4 alike) : Display
  Ground_2 : Ground
  Ground_3 : Ground
  Ground_4 : Ground
  MuxState : Subsystem  Tag=mux/State  mask(Empty Dynamics State Block){positioningmode=on, TimeStep=1/20}
      mask prompts: positioningmode "Positioning Mode"; TimeStep "Auto Assigned: Time Step [s]"
      mask help:
      | Build the state of an actor based on user input.
      | The user can either use positioning mode or dynamics mode.
      | - When using positioning mode the position and orientation of the actor are set directly based on the input. Expected input is relative to the initial position and orientation of the actor. It's also possible to specify the velocity of the actor, though this input isn't used, only passed on.
      | - When using dynamics mode the position input is ignored. Expected input is velocity and orientation. The velocity is relative the current orientation of the actor, while orientation is relative to its initial orientation. The position of the actor is calculated based on the velocity and orientation given.
      settings: DeleteFcn=PreScanBlockDeleteFcn;
  STATE_Male_Overweight_1 : Subsystem  Tag=mux/StatePort  Priority=0  LoadFcn=load PrescanStateActuatorData  mask(PreScan Sink Block: State){x0=W01_Base_Map_cs_44df0411d70deda6, y0=W01_Base_Map_cs_f2ae0dab17c72fbc, z0=W01_Base_Map_cs_8c8b17a14e31d025, Roll0=W01_Base_Map_cs_0a863e6a78242047, Pitch0=W01_Base_Map_cs_30b59f3a412629bc, Yaw0=W01_Base_Map_cs_b74abb8bb5ceb81f, TimeStep=1/20}
      mask prompts: x0 "Ini x-position VEHICLE wrt GLOBAL axis system [m]"; y0 "Ini y-position VEHICLE wrt GLOBAL axis system [m]"; z0 "Ini z-position VEHICLE wrt GLOBAL axis system [m]"; Roll0 "Ini roll-angle BODY wrt VEHICLE axis system [deg]"; Pitch0 "Ini pitch-angle BODY wrt VEHICLE axis system [deg]"; Yaw0 "Ini yaw-angle VEHICLE wrt GLOBAL axis system [deg]"; TimeStep "Auto-Assigned: Upload Period [s]"
      mask help:
      | The Actor State contains a vector signal of size (9x1), containing the following signals:
      |
      | -  Position                  (x,y,z)                                     [m]
      | -  Velocity                  (vx,vy,vz)                               [m/s]
      | -  Angles                    (Roll, Pitch, Yaw)                   [rad]
      |
      | The Actor state is defined in the global axis system.
      | The state is superponed on the Initial position defined in the GUI.
      |
      | For more information, please click Help.
      settings: DeleteFcn=PreScanBlockDeleteFcn;
      mask Help: eval('openHelp(222)')
      mask Display: image(imread('State.png'))
  To Virtual Bus : SignalConversion  ConversionOutput=Virtual bus  OverrideOpt=off
  State : Outport  Tag=outport/StateOutport  SampleTime=1/20
  wires:
  MuxState/1(state) -> STATE_Male_Overweight_1/1(State)
  STATE_Male_Overweight_1/1(StateBus) -> State/1
  Ground_2/1 -> MuxState/4(dx [m/s])
  Ground_3/1 -> MuxState/5(dy [m/s])
  Ground_4/1 -> MuxState/6(dz [m/s])
  Bus Selector/2 -> MuxState/8(P [rad]), Display/1  "<signal2>"
  Bus Selector/1 -> MuxState/7(R [rad]), Display2/1  "<signal1>"
  Bus Selector1/2 -> MuxState/2(y [m])  "<Y>"
  Bus Selector1/1 -> MuxState/1(x [m])  "<X>"
  Coordinate Transformation Conversion/1 -> Demux/1
  Demux/1 -> Bus Creator/1
  To Virtual Bus/1 -> Bus to Vector/1
  In1/1 -> Bus Selector1/1
  Bus to Vector/1 -> Display3/1, Coordinate Transformation Conversion/1
  Bus Creator1/1 -> To Virtual Bus/1
  Demux/2 -> Bus Creator/2
  Demux/3 -> Bus Creator/3
  Bus Creator/1 -> Bus Selector/1
  Bus Selector1/7 -> Bus Creator1/4  "<Z>"
  Bus Selector1/4 -> Bus Creator1/1  "<W>"
  Bus Selector/3 -> MuxState/9(Y [rad]), Display1/1  "<signal3>"
  Bus Selector1/5 -> Bus Creator1/2  "<X>"
  Bus Selector1/3 -> MuxState/3(z [m])  "<Z>"
  Bus Selector1/6 -> Bus Creator1/3  "<Y>"

== system W01_Base_Map_cs/Male_Overweight_1/SELF_Demux ==
  SELF : Inport  OutDataTypeStr=Bus: PRESCAN_SELFSENSORDATA
  Bus Selector : BusSelector  OutputSignals=PositionX,PositionY,PositionZ,OrientationRoll,OrientationPitch,OrientationYaw,Velocity,Yaw_rate,Lat,Long,Alt,TimeStamp
  Demux2 : Demux  Outputs=3
  Gain : Gain  Gain=180/pi
  Gain1 : Gain  Gain=180/pi
  Vector Concatenate1 : Concatenate  NumInputs=3
  compas converter : Subsystem
  x [m] : Outport
  y [m] : Outport  Port=2
  z [m] : Outport  Port=3
  rotx [deg] : Outport  Port=4
  roty [deg] : Outport  Port=5
  rotz [deg] : Outport  Port=6
  GPS lat [deg] : Outport  Port=7
  GPS long [deg] : Outport  Port=8
  GPS alt [m] : Outport  Port=9
  velocity [m/s] : Outport  Port=10
  heading [deg] : Outport  Port=11
  yaw rate [deg/s] : Outport  Port=12
  TimeStamp [s] : Outport  Port=13
  wires:
  Bus Selector/12 -> TimeStamp [s]/1  "<TimeStamp>"
  Bus Selector/11 -> GPS alt [m]/1  "<Alt>"
  Bus Selector/10 -> GPS long [deg]/1  "<Long>"
  Bus Selector/9 -> GPS lat [deg]/1  "<Lat>"
  Bus Selector/8 -> Gain1/1  "<Yaw_rate>"
  Bus Selector/7 -> velocity [m/s]/1  "<Velocity>"
  Bus Selector/6 -> compas converter/1(rotz [rad]), Vector Concatenate1/3  "<OrientationYaw>"
  Bus Selector/5 -> Vector Concatenate1/2  "<OrientationPitch>"
  Bus Selector/4 -> Vector Concatenate1/1  "<OrientationRoll>"
  Vector Concatenate1/1 -> Gain/1
  Bus Selector/3 -> z [m]/1  "<PositionZ>"
  Bus Selector/2 -> y [m]/1  "<PositionY>"
  Bus Selector/1 -> x [m]/1  "<PositionX>"
  SELF/1 -> Bus Selector/1
  Gain/1 -> Demux2/1
  Demux2/1 -> rotx [deg]/1
  Demux2/2 -> roty [deg]/1
  Demux2/3 -> rotz [deg]/1
  compas converter/1(heading [deg]) -> heading [deg]/1
  Gain1/1 -> yaw rate [deg/s]/1

== system W01_Base_Map_cs/Male_Overweight_1/VISUColorRegion_Lower_Body_Mux ==
  RGB [-,-,-] : Inport
  Bus Creator : BusCreator  Inputs=4  OutDataTypeStr=Bus: PRESCAN_COLOR_DATA  NonVirtualBus=on
  Constant : Constant  Value=255  OutDataTypeStr=uint8
  Data Type Conversion : DataTypeConversion  OutDataTypeStr=uint8
  Data Type Conversion1 : DataTypeConversion  OutDataTypeStr=uint8
  Data Type Conversion2 : DataTypeConversion  OutDataTypeStr=uint8
  Demux : Demux  Outputs=3
  ColorRegion : Outport  OutDataTypeStr=Bus: PRESCAN_COLOR_DATA  PortDimensions=1
  wires:
  Constant/1 -> Bus Creator/4  "A"
  Data Type Conversion2/1 -> Bus Creator/3  "B"
  Data Type Conversion1/1 -> Bus Creator/2  "G"
  Data Type Conversion/1 -> Bus Creator/1  "R"
  Demux/3 -> Data Type Conversion2/1  "B"
  Demux/2 -> Data Type Conversion1/1  "G"
  Demux/1 -> Data Type Conversion/1  "R"
  RGB [-,-,-]/1 -> Demux/1
  Bus Creator/1 -> ColorRegion/1

== system W01_Base_Map_cs/Male_Overweight_1/VISUColorRegion_Shoes_Mux ==
  RGB [-,-,-] : Inport
  Bus Creator : BusCreator  Inputs=4  OutDataTypeStr=Bus: PRESCAN_COLOR_DATA  NonVirtualBus=on
  Constant : Constant  Value=255  OutDataTypeStr=uint8
  Data Type Conversion : DataTypeConversion  OutDataTypeStr=uint8
  Data Type Conversion1 : DataTypeConversion  OutDataTypeStr=uint8
  Data Type Conversion2 : DataTypeConversion  OutDataTypeStr=uint8
  Demux : Demux  Outputs=3
  ColorRegion : Outport  OutDataTypeStr=Bus: PRESCAN_COLOR_DATA  PortDimensions=1
  wires:
  Constant/1 -> Bus Creator/4  "A"
  Data Type Conversion2/1 -> Bus Creator/3  "B"
  Data Type Conversion1/1 -> Bus Creator/2  "G"
  Data Type Conversion/1 -> Bus Creator/1  "R"
  Demux/3 -> Data Type Conversion2/1  "B"
  Demux/2 -> Data Type Conversion1/1  "G"
  Demux/1 -> Data Type Conversion/1  "R"
  RGB [-,-,-]/1 -> Demux/1
  Bus Creator/1 -> ColorRegion/1

== system W01_Base_Map_cs/Male_ShoppingBag_1/Animation ==
  In1 : Inport
  Bus Creator : BusCreator  Inputs=2  OutDataTypeStr=Bus: PRESCAN_ANIMACTUATORDATA  NonVirtualBus=on
  Bus Selector : BusSelector  OutputSignals=VelocityX,VelocityY,VelocityZ
  Mux : Mux  Inputs=3
  animation mode : Subsystem
  elapsed track : Subsystem
  Out1 : Outport
  wires:
  animation mode/1(mode) -> Bus Creator/1  "Index"
  Bus Creator/1 -> Out1/1
  In1/1 -> Bus Selector/1
  elapsed track/1(s) -> Bus Creator/2  "Time"
  Bus Selector/3 -> Mux/3  "<VelocityZ>"
  Bus Selector/2 -> Mux/2  "<VelocityY>"
  Bus Selector/1 -> Mux/1  "<VelocityX>"
  Mux/1 -> animation mode/1(vel), elapsed track/1(vel)

== system W01_Base_Map_cs/Male_ShoppingBag_1/Dynamics_Empty ==
  note: For state mode 'Dynamic' positions
      | are not taken into account, as they
      | are computed by integrating velocity.
      | Click annotation for Help.
  In1 : Inport
  Bus Creator : BusCreator  Inputs=3
  Bus Creator1 : BusCreator  Inputs=4
  Bus Selector : BusSelector  OutputSignals=signal1,signal2,signal3
  Bus Selector1 : BusSelector  OutputSignals=Pose.Position.X,Pose.Position.Y,Pose.Position.Z,Pose.Orientation.W,Pose.Orientation.X,Pose.Orientation.Y,Pose.Orientation.Z
  Bus to Vector : BusToVector
  Coordinate Transformation Conversion : robotcorelib/Coordinate Transformation Conversion  InputRepresentation=Quaternion  InputEulerSequence=ZYX  ShowTrVecInputPort=on  OutputRepresentation=Euler Angles  OutputEulerSequence=ZYX  ShowTrVecOutputPort=on  SimulateUsing=Interpreted execution
      settings: SourceProductBaseCode=RO
  Demux : Demux  Outputs=3
  Display{,1..3} (4 alike) : Display
  Ground_2 : Ground
  Ground_3 : Ground
  Ground_4 : Ground
  MuxState : Subsystem  Tag=mux/State  mask(Empty Dynamics State Block){positioningmode=on, TimeStep=1/20}
      mask prompts: positioningmode "Positioning Mode"; TimeStep "Auto Assigned: Time Step [s]"
      mask help:
      | Build the state of an actor based on user input.
      | The user can either use positioning mode or dynamics mode.
      | - When using positioning mode the position and orientation of the actor are set directly based on the input. Expected input is relative to the initial position and orientation of the actor. It's also possible to specify the velocity of the actor, though this input isn't used, only passed on.
      | - When using dynamics mode the position input is ignored. Expected input is velocity and orientation. The velocity is relative the current orientation of the actor, while orientation is relative to its initial orientation. The position of the actor is calculated based on the velocity and orientation given.
      settings: DeleteFcn=PreScanBlockDeleteFcn;
  STATE_Male_ShoppingBag_1 : Subsystem  Tag=mux/StatePort  Priority=0  LoadFcn=load PrescanStateActuatorData  mask(PreScan Sink Block: State){x0=W01_Base_Map_cs_b6f9a9d42e1fb114, y0=W01_Base_Map_cs_291a12e3480490a5, z0=W01_Base_Map_cs_adbbd85f61202ab7, Roll0=W01_Base_Map_cs_4a768cb681f8a4c2, Pitch0=W01_Base_Map_cs_d74a044cdf4d1848, Yaw0=W01_Base_Map_cs_f2c5778ca349af40, TimeStep=1/20}
      mask prompts: x0 "Ini x-position VEHICLE wrt GLOBAL axis system [m]"; y0 "Ini y-position VEHICLE wrt GLOBAL axis system [m]"; z0 "Ini z-position VEHICLE wrt GLOBAL axis system [m]"; Roll0 "Ini roll-angle BODY wrt VEHICLE axis system [deg]"; Pitch0 "Ini pitch-angle BODY wrt VEHICLE axis system [deg]"; Yaw0 "Ini yaw-angle VEHICLE wrt GLOBAL axis system [deg]"; TimeStep "Auto-Assigned: Upload Period [s]"
      mask help:
      | The Actor State contains a vector signal of size (9x1), containing the following signals:
      |
      | -  Position                  (x,y,z)                                     [m]
      | -  Velocity                  (vx,vy,vz)                               [m/s]
      | -  Angles                    (Roll, Pitch, Yaw)                   [rad]
      |
      | The Actor state is defined in the global axis system.
      | The state is superponed on the Initial position defined in the GUI.
      |
      | For more information, please click Help.
      settings: DeleteFcn=PreScanBlockDeleteFcn;
      mask Help: eval('openHelp(222)')
      mask Display: image(imread('State.png'))
  To Virtual Bus : SignalConversion  ConversionOutput=Virtual bus  OverrideOpt=off
  State : Outport  Tag=outport/StateOutport  SampleTime=1/20
  wires:
  MuxState/1(state) -> STATE_Male_ShoppingBag_1/1(State)
  STATE_Male_ShoppingBag_1/1(StateBus) -> State/1
  Ground_2/1 -> MuxState/4(dx [m/s])
  Ground_3/1 -> MuxState/5(dy [m/s])
  Ground_4/1 -> MuxState/6(dz [m/s])
  Coordinate Transformation Conversion/1 -> Demux/1
  Demux/1 -> Bus Creator/1
  To Virtual Bus/1 -> Bus to Vector/1
  Bus to Vector/1 -> Display3/1, Coordinate Transformation Conversion/1
  Bus Creator1/1 -> To Virtual Bus/1
  Demux/2 -> Bus Creator/2
  Demux/3 -> Bus Creator/3
  Bus Creator/1 -> Bus Selector/1
  Bus Selector1/7 -> Bus Creator1/4  "<Z>"
  Bus Selector1/4 -> Bus Creator1/1  "<W>"
  Bus Selector1/5 -> Bus Creator1/2  "<X>"
  Bus Selector1/6 -> Bus Creator1/3  "<Y>"
  In1/1 -> Bus Selector1/1
  Bus Selector1/1 -> MuxState/1(x [m])  "<X>"
  Bus Selector1/2 -> MuxState/2(y [m])  "<Y>"
  Bus Selector1/3 -> MuxState/3(z [m])  "<Z>"
  Bus Selector/1 -> Display2/1, MuxState/7(R [rad])  "<signal1>"
  Bus Selector/2 -> Display/1, MuxState/8(P [rad])  "<signal2>"
  Bus Selector/3 -> Display1/1, MuxState/9(Y [rad])  "<signal3>"

== system W01_Base_Map_cs/Male_ShoppingBag_1/SELF_Demux ==
  SELF : Inport  OutDataTypeStr=Bus: PRESCAN_SELFSENSORDATA
  Bus Selector : BusSelector  OutputSignals=PositionX,PositionY,PositionZ,OrientationRoll,OrientationPitch,OrientationYaw,Velocity,Yaw_rate,Lat,Long,Alt,TimeStamp
  Demux2 : Demux  Outputs=3
  Gain : Gain  Gain=180/pi
  Gain1 : Gain  Gain=180/pi
  Vector Concatenate1 : Concatenate  NumInputs=3
  compas converter : Subsystem
  x [m] : Outport
  y [m] : Outport  Port=2
  z [m] : Outport  Port=3
  rotx [deg] : Outport  Port=4
  roty [deg] : Outport  Port=5
  rotz [deg] : Outport  Port=6
  GPS lat [deg] : Outport  Port=7
  GPS long [deg] : Outport  Port=8
  GPS alt [m] : Outport  Port=9
  velocity [m/s] : Outport  Port=10
  heading [deg] : Outport  Port=11
  yaw rate [deg/s] : Outport  Port=12
  TimeStamp [s] : Outport  Port=13
  wires:
  Bus Selector/12 -> TimeStamp [s]/1  "<TimeStamp>"
  Bus Selector/11 -> GPS alt [m]/1  "<Alt>"
  Bus Selector/10 -> GPS long [deg]/1  "<Long>"
  Bus Selector/9 -> GPS lat [deg]/1  "<Lat>"
  Bus Selector/8 -> Gain1/1  "<Yaw_rate>"
  Bus Selector/7 -> velocity [m/s]/1  "<Velocity>"
  Bus Selector/6 -> compas converter/1(rotz [rad]), Vector Concatenate1/3  "<OrientationYaw>"
  Bus Selector/5 -> Vector Concatenate1/2  "<OrientationPitch>"
  Bus Selector/4 -> Vector Concatenate1/1  "<OrientationRoll>"
  Vector Concatenate1/1 -> Gain/1
  Bus Selector/3 -> z [m]/1  "<PositionZ>"
  Bus Selector/2 -> y [m]/1  "<PositionY>"
  Bus Selector/1 -> x [m]/1  "<PositionX>"
  SELF/1 -> Bus Selector/1
  Gain/1 -> Demux2/1
  Demux2/1 -> rotx [deg]/1
  Demux2/2 -> roty [deg]/1
  Demux2/3 -> rotz [deg]/1
  compas converter/1(heading [deg]) -> heading [deg]/1
  Gain1/1 -> yaw rate [deg/s]/1

== system W01_Base_Map_cs/Male_ShoppingBag_1/VISUColorRegion_Bag_Mux ==
  RGB [-,-,-] : Inport
  Bus Creator : BusCreator  Inputs=4  OutDataTypeStr=Bus: PRESCAN_COLOR_DATA  NonVirtualBus=on
  Constant : Constant  Value=255  OutDataTypeStr=uint8
  Data Type Conversion : DataTypeConversion  OutDataTypeStr=uint8
  Data Type Conversion1 : DataTypeConversion  OutDataTypeStr=uint8
  Data Type Conversion2 : DataTypeConversion  OutDataTypeStr=uint8
  Demux : Demux  Outputs=3
  ColorRegion : Outport  OutDataTypeStr=Bus: PRESCAN_COLOR_DATA  PortDimensions=1
  wires:
  Constant/1 -> Bus Creator/4  "A"
  Data Type Conversion2/1 -> Bus Creator/3  "B"
  Data Type Conversion1/1 -> Bus Creator/2  "G"
  Data Type Conversion/1 -> Bus Creator/1  "R"
  Demux/3 -> Data Type Conversion2/1  "B"
  Demux/2 -> Data Type Conversion1/1  "G"
  Demux/1 -> Data Type Conversion/1  "R"
  RGB [-,-,-]/1 -> Demux/1
  Bus Creator/1 -> ColorRegion/1

== system W01_Base_Map_cs/Male_ShoppingBag_1/VISUColorRegion_Lower_Body_Mux ==
  RGB [-,-,-] : Inport
  Bus Creator : BusCreator  Inputs=4  OutDataTypeStr=Bus: PRESCAN_COLOR_DATA  NonVirtualBus=on
  Constant : Constant  Value=255  OutDataTypeStr=uint8
  Data Type Conversion : DataTypeConversion  OutDataTypeStr=uint8
  Data Type Conversion1 : DataTypeConversion  OutDataTypeStr=uint8
  Data Type Conversion2 : DataTypeConversion  OutDataTypeStr=uint8
  Demux : Demux  Outputs=3
  ColorRegion : Outport  OutDataTypeStr=Bus: PRESCAN_COLOR_DATA  PortDimensions=1
  wires:
  Constant/1 -> Bus Creator/4  "A"
  Data Type Conversion2/1 -> Bus Creator/3  "B"
  Data Type Conversion1/1 -> Bus Creator/2  "G"
  Data Type Conversion/1 -> Bus Creator/1  "R"
  Demux/3 -> Data Type Conversion2/1  "B"
  Demux/2 -> Data Type Conversion1/1  "G"
  Demux/1 -> Data Type Conversion/1  "R"
  RGB [-,-,-]/1 -> Demux/1
  Bus Creator/1 -> ColorRegion/1
